simulink model "hw2"  (R2024a)
settings: Solver=VariableStepAuto  StartTime=0.0  StopTime=100  RelTol=1e-3
settings Model: Creator=mrdan  LastModifiedBy=mrdan

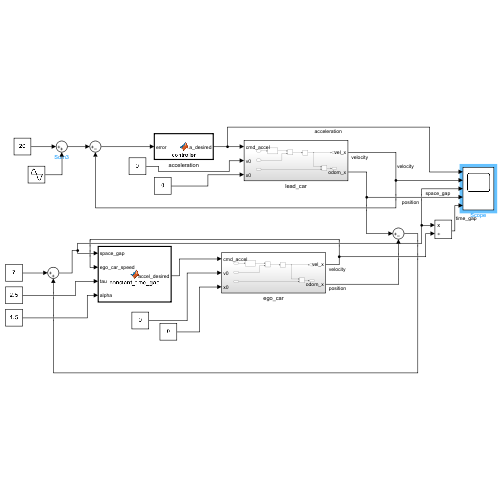
[thumbnail: Simulink's stored preview of the top-level diagram]
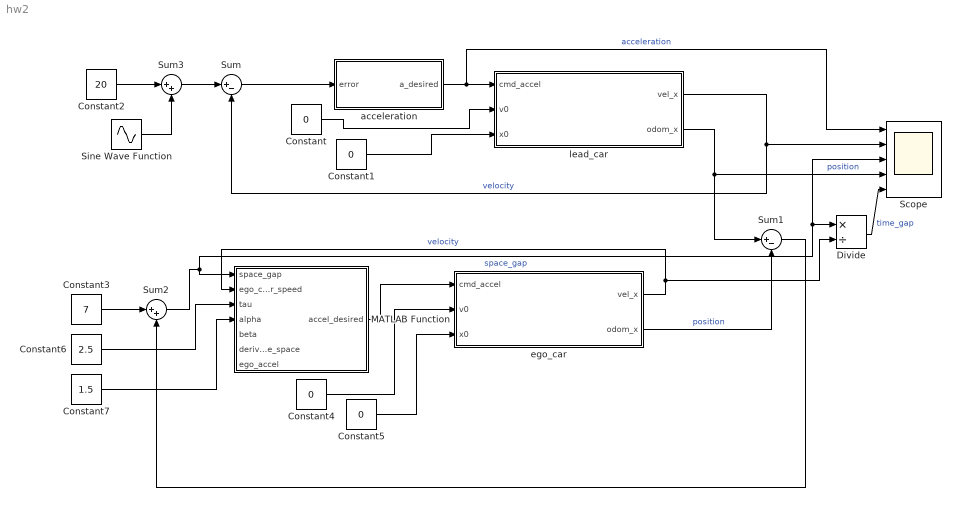
== system hw2 ==
  Constant{,1,4..5} (4 alike) : Constant  Value=0
  Constant2 : Constant  Value=20
  Constant3 : Constant  Value=7
  Constant6 : Constant  Value=2.5
  Constant7 : Constant  Value=1.5
  Divide : Product  Inputs=*/
  MATLAB Function : MATLAB Function  TreatAsAtomicUnit=on
  Scope : Scope  NumInputPorts=5
  Sine Wave Function : Sin  Amplitude=5  SampleTime=0
  Sum : Sum  Inputs=|+-
  Sum1 : Sum  Inputs=|+-
  Sum2 : Sum  Inputs=|++
  Sum3 : Sum  Inputs=|++
  acceleration : MATLAB Function  TreatAsAtomicUnit=on
  ego_car : Subsystem
  lead_car : Subsystem
  wires:
  acceleration/1(a_desired) -> Scope/1, lead_car/1(cmd_accel)  "acceleration"
  Sum/1 -> acceleration/1(error)
  lead_car/2(odom_x) -> Sum1/1, Scope/4  "position"
  Constant1/1 -> lead_car/3(x0)
  Constant/1 -> lead_car/2(v0)
  lead_car/1(vel_x) -> Sum/2, Scope/2  "velocity"
  Constant3/1 -> Sum2/1
  Sum1/1 -> Sum2/2
  Sum2/1 -> Divide/1, Scope/3, MATLAB Function/1(space_gap)  "space_gap"
  MATLAB Function/1(accel_desired) -> ego_car/1(cmd_accel)
  Constant4/1 -> ego_car/2(v0)
  Constant5/1 -> ego_car/3(x0)
  ego_car/2(odom_x) -> Sum1/2  "position"
  ego_car/1(vel_x) -> MATLAB Function/2(ego_car_speed), Divide/2  "velocity"
  Constant6/1 -> MATLAB Function/3(tau)
  Constant7/1 -> MATLAB Function/4(alpha)
  Constant2/1 -> Sum3/1
  Sine Wave Function/1 -> Sum3/2
  Sum3/1 -> Sum/1
  Divide/1 -> Scope/5  "time_gap"

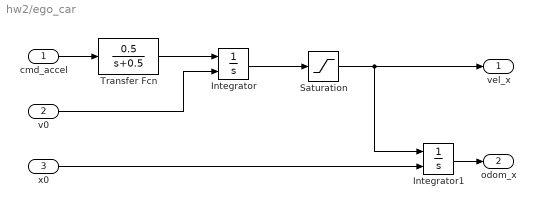
== system hw2/ego_car ==
  cmd_accel : Inport
  v0 : Inport  Port=2
  x0 : Inport  Port=3
  Integrator : Integrator  InitialConditionSource=external
  Integrator1 : Integrator  InitialConditionSource=external
  Saturation : Saturate  UpperLimit=80  LowerLimit=0
  Transfer Fcn : TransferFcn  Numerator=[0.5]  Denominator=[1 0.5]
  vel_x : Outport
  odom_x : Outport  Port=2
  wires:
  v0/1 -> Integrator/2
  cmd_accel/1 -> Transfer Fcn/1
  Transfer Fcn/1 -> Integrator/1
  Integrator1/1 -> odom_x/1
  Integrator/1 -> Saturation/1
  x0/1 -> Integrator1/2
  Saturation/1 -> vel_x/1, Integrator1/1

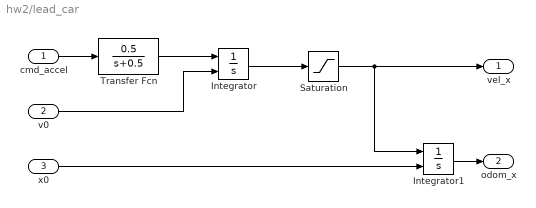
== system hw2/lead_car ==
  cmd_accel : Inport
  v0 : Inport  Port=2
  x0 : Inport  Port=3
  Integrator : Integrator  InitialConditionSource=external
  Integrator1 : Integrator  InitialConditionSource=external
  Saturation : Saturate  UpperLimit=80  LowerLimit=0
  Transfer Fcn : TransferFcn  Numerator=[0.5]  Denominator=[1 0.5]
  vel_x : Outport
  odom_x : Outport  Port=2
  wires:
  v0/1 -> Integrator/2
  cmd_accel/1 -> Transfer Fcn/1
  Transfer Fcn/1 -> Integrator/1
  Integrator1/1 -> odom_x/1
  Integrator/1 -> Saturation/1
  x0/1 -> Integrator1/2
  Saturation/1 -> vel_x/1, Integrator1/1

== matlab function hw2/MATLAB Function ==
  data: space_gap input; accel_desired output; ego_car_speed input; tau input; alpha input; beta input; derivative_space input; ego_accel input
function accel_desired = constant_time_gap(space_gap, ego_car_speed, tau, alpha, beta, derivative_space, ego_accel)

accel_desired = alpha * (space_gap - tau * ego_car_speed) + beta * (derivative_space - tau * ego_accel);

== matlab function hw2/acceleration ==
  data: error input; a_desired output
function a_desired = controller(error)
a_desired = max(-1.5, min(3, error));
end
